simulink model "Tipo4_v4"  (R2018b)
settings: Solver=FixedStepDiscrete  StartTime=0.0  StopTime=50.3  MaxStep=50e-6  RelTol=1e-3
PreLoadFcn:
  | Ts=2e-6;
InitFcn:
  | %xInitial = init_power_wind_dfig_det;
  | Ts=2e-6;
undefined symbols (not defined in the file): D1, Delta, DiscIntNeverNeededParam, find_system
libraries: powerlib x144, simulink x110, powerlib_meascontrol x83, simulink_extras x6, powerlib_extras x4
(part 4 of 6)

== system Tipo4_v4/Subsystem7 ==
  In1 : Inport
  Bistable{,1..3} (4 alike) : powerlib_meascontrol/Logic/Bistable  Qpriority=Set  ic=0  Ts=Ts
      settings: SourceProductName=Simscape Power Systems  SourceProductBaseCode=PS
  Clock{,1..3} (4 alike) : Clock
  Compare To Constant{,2,4,6} (4 alike) : simulink/Logic and Bit Operations/Compare To Constant  relop=<=  const=100  OutDataTypeStr=uint8
  Compare To Constant1 : simulink/Logic and Bit Operations/Compare To Constant  relop=>=  const=Tini_FT  OutDataTypeStr=uint8
  Compare To Constant3 : simulink/Logic and Bit Operations/Compare To Constant  relop=>=  const=Tini_FF  OutDataTypeStr=uint8
  Compare To Constant5 : simulink/Logic and Bit Operations/Compare To Constant  relop=>=  const=Tini_FFT  OutDataTypeStr=uint8
  Compare To Constant7 : simulink/Logic and Bit Operations/Compare To Constant  relop=>=  const=Tini_FFF  OutDataTypeStr=uint8
  Compare To Constant8 : simulink/Logic and Bit Operations/Compare To Constant  relop=<=  const=0.1*pi/180  OutDataTypeStr=uint8
  Constant : Constant  Value=Tini_FT
  Constant1 : Constant  Value=Tini_FF
  Constant2 : Constant  Value=Tini_FFT
  Constant3 : Constant  Value=Tini_FFF
  Gain{,1..3} (4 alike) : Gain  OutDataTypeStr=double
  Ground : powerlib/Elements/Ground  LConnTagsString=a
  Ground1 : powerlib/Elements/Ground  LConnTagsString=a
  Ground2 : powerlib/Elements/Ground  LConnTagsString=a
  Mux1 : Mux  Inputs=3
  PLL (3ph) : powerlib_meascontrol/PLL/PLL (3ph)  Fmin=60  Par_Init=[0, 60]  ParK=[180, 3200, 1]  TcD=1e-4  MaxRateChangeFreq=12  FilterCutOffFreq=25  Ts=Ts  AGC=on
  Product{,2..7} (7 alike) : Product
  Product{1,8..11} (5 alike) : Product  RndMeth=Ceiling
  Scope{1..4} (4 alike) : Scope
  Three-Phase Fault1 : powerlib/Elements/Three-Phase Fault  InitialStates=0  FaultA=on  FaultB=off  FaultC=off  GroundFault=on  SwitchTimes=[900 1000]  External=on  SwitchStatus=NaN  FaultResistance=R_falta  GroundResistance=R_falta  SnubberResistance=1e6  SnubberCapacitance=inf  Measurements=None
  Three-Phase Fault2 : powerlib/Elements/Three-Phase Fault  InitialStates=0  FaultA=on  FaultB=on  FaultC=off  GroundFault=off  SwitchTimes=[900 1000]  External=on  SwitchStatus=NaN  FaultResistance=R_falta  GroundResistance=1e-12  SnubberResistance=1e6  SnubberCapacitance=inf  Measurements=None
  Three-Phase Fault3 : powerlib/Elements/Three-Phase Fault  InitialStates=0  FaultA=on  FaultB=on  FaultC=off  GroundFault=on  SwitchTimes=[900 1000]  External=on  SwitchStatus=NaN  FaultResistance=R_falta  GroundResistance=R_falta  SnubberResistance=1e6  SnubberCapacitance=inf  Measurements=None
  Three-Phase Fault4 : powerlib/Elements/Three-Phase Fault  InitialStates=0  FaultA=on  FaultB=on  FaultC=on  GroundFault=on  SwitchTimes=[900 1000]  External=on  SwitchStatus=NaN  FaultResistance=R_falta  GroundResistance=R_falta  SnubberResistance=1e6  SnubberCapacitance=inf  Measurements=None
  Voltage Measurement : powerlib/Measurements/Voltage Measurement  PhasorSimulation=off  OutputType=Complex  PSBequivalent=0
  Voltage Measurement1 : powerlib/Measurements/Voltage Measurement  PhasorSimulation=off  OutputType=Complex  PSBequivalent=0
  Voltage Measurement2 : powerlib/Measurements/Voltage Measurement  PhasorSimulation=off  OutputType=Complex  PSBequivalent=0
  A : PMIOPort  Tag=PMCPort  Side=Right
  B : PMIOPort  Tag=PMCPort  Port=2  Side=Right
  C : PMIOPort  Tag=PMCPort  Port=3  Side=Right
  wires:
  Clock/1 -> Compare To Constant1/1
  Product2/1 -> Product3/1
  Constant1/1 -> Compare To Constant2/1
  Product/1 -> Product1/1
  Compare To Constant2/1 -> Product2/2
  Constant2/1 -> Compare To Constant4/1
  Clock2/1 -> Compare To Constant5/1
  Compare To Constant4/1 -> Product4/2
  Clock1/1 -> Compare To Constant3/1
  Compare To Constant5/1 -> Product5/2
  In1/1 -> Product/1, Product2/1, Product4/1, Product6/1
  Clock3/1 -> Compare To Constant7/1
  Constant3/1 -> Compare To Constant6/1
  Compare To Constant6/1 -> Product6/2
  Product6/1 -> Product7/1
  Compare To Constant7/1 -> Product7/2
  Compare To Constant3/1 -> Product3/2
  Constant/1 -> Compare To Constant/1
  Compare To Constant/1 -> Product/2
  Compare To Constant1/1 -> Product1/2
  Product4/1 -> Product5/1
  Product1/1 -> Product8/2
  Product8/1 -> Bistable/1
  Product3/1 -> Product9/2
  Product5/1 -> Product10/2
  Product7/1 -> Product11/2
  Compare To Constant8/1 -> Product11/1, Product10/1, Product9/1, Product8/1
  PLL (3ph)/2 -> Compare To Constant8/1
  Voltage Measurement1/1 -> Mux1/2
  Voltage Measurement/1 -> Mux1/1
  Voltage Measurement2/1 -> Mux1/3
  Mux1/1 -> PLL (3ph)/1
  Gain/1 -> Scope1/1, Three-Phase Fault1/1
  Gain1/1 -> Scope2/1, Three-Phase Fault2/1
  Gain2/1 -> Three-Phase Fault3/1, Scope3/1
  Gain3/1 -> Scope4/1, Three-Phase Fault4/1
  Bistable/1 -> Gain/1
  Product9/1 -> Bistable1/1
  Bistable1/1 -> Gain1/1
  Bistable3/1 -> Gain2/1
  Product10/1 -> Bistable3/1
  Product11/1 -> Bistable2/1
  Bistable2/1 -> Gain3/1
  connections:
  Voltage Measurement1/LConn1 -- B/RConn1 -- Three-Phase Fault1/LConn2 -- Three-Phase Fault2/LConn2 -- Three-Phase Fault3/LConn2 -- Three-Phase Fault4/LConn2
  Voltage Measurement2/LConn1 -- C/RConn1 -- Three-Phase Fault4/LConn3 -- Three-Phase Fault3/LConn3 -- Three-Phase Fault2/LConn3 -- Three-Phase Fault1/LConn3
  A/RConn1 -- Voltage Measurement/LConn1 -- Three-Phase Fault1/LConn1 -- Three-Phase Fault2/LConn1 -- Three-Phase Fault3/LConn1 -- Three-Phase Fault4/LConn1
  Ground/LConn1 -- Voltage Measurement/LConn2
  Ground1/LConn1 -- Voltage Measurement1/LConn2
  Ground2/LConn1 -- Voltage Measurement2/LConn2

== system Tipo4_v4/Subsystem8 ==
  In1 : Inport
  Bistable{,1..3} (4 alike) : powerlib_meascontrol/Logic/Bistable  Qpriority=Set  ic=0  Ts=Ts
      settings: SourceProductName=Simscape Power Systems  SourceProductBaseCode=PS
  Clock{,1..3} (4 alike) : Clock
  Compare To Constant{,2,4,6} (4 alike) : simulink/Logic and Bit Operations/Compare To Constant  relop=<=  const=100  OutDataTypeStr=uint8
  Compare To Constant1 : simulink/Logic and Bit Operations/Compare To Constant  relop=>=  const=Tini_FT  OutDataTypeStr=uint8
  Compare To Constant3 : simulink/Logic and Bit Operations/Compare To Constant  relop=>=  const=Tini_FF  OutDataTypeStr=uint8
  Compare To Constant5 : simulink/Logic and Bit Operations/Compare To Constant  relop=>=  const=Tini_FFT  OutDataTypeStr=uint8
  Compare To Constant7 : simulink/Logic and Bit Operations/Compare To Constant  relop=>=  const=Tini_FFF  OutDataTypeStr=uint8
  Compare To Constant8 : simulink/Logic and Bit Operations/Compare To Constant  relop=<=  const=0.1*pi/180  OutDataTypeStr=uint8
  Constant : Constant  Value=Tini_FT
  Constant1 : Constant  Value=Tini_FF
  Constant2 : Constant  Value=Tini_FFT
  Constant3 : Constant  Value=Tini_FFF
  Gain{,1..3} (4 alike) : Gain  OutDataTypeStr=double
  Ground : powerlib/Elements/Ground  LConnTagsString=a
  Ground1 : powerlib/Elements/Ground  LConnTagsString=a
  Ground2 : powerlib/Elements/Ground  LConnTagsString=a
  Mux1 : Mux  Inputs=3
  PLL (3ph) : powerlib_meascontrol/PLL/PLL (3ph)  Fmin=60  Par_Init=[0, 60]  ParK=[180, 3200, 1]  TcD=1e-4  MaxRateChangeFreq=12  FilterCutOffFreq=25  Ts=Ts  AGC=on
  Product{,2..7} (7 alike) : Product
  Product{1,8..11} (5 alike) : Product  RndMeth=Ceiling
  Scope{1..4} (4 alike) : Scope
  Three-Phase Fault1 : powerlib/Elements/Three-Phase Fault  InitialStates=0  FaultA=on  FaultB=off  FaultC=off  GroundFault=on  SwitchTimes=[900 1000]  External=on  SwitchStatus=NaN  FaultResistance=R_falta  GroundResistance=R_falta  SnubberResistance=1e6  SnubberCapacitance=inf  Measurements=None
  Three-Phase Fault2 : powerlib/Elements/Three-Phase Fault  InitialStates=0  FaultA=on  FaultB=on  FaultC=off  GroundFault=off  SwitchTimes=[900 1000]  External=on  SwitchStatus=NaN  FaultResistance=R_falta  GroundResistance=1e-12  SnubberResistance=1e6  SnubberCapacitance=inf  Measurements=None
  Three-Phase Fault3 : powerlib/Elements/Three-Phase Fault  InitialStates=0  FaultA=on  FaultB=on  FaultC=off  GroundFault=on  SwitchTimes=[900 1000]  External=on  SwitchStatus=NaN  FaultResistance=R_falta  GroundResistance=R_falta  SnubberResistance=1e6  SnubberCapacitance=inf  Measurements=None
  Three-Phase Fault4 : powerlib/Elements/Three-Phase Fault  InitialStates=0  FaultA=on  FaultB=on  FaultC=on  GroundFault=on  SwitchTimes=[900 1000]  External=on  SwitchStatus=NaN  FaultResistance=R_falta  GroundResistance=R_falta  SnubberResistance=1e6  SnubberCapacitance=inf  Measurements=None
  Voltage Measurement : powerlib/Measurements/Voltage Measurement  PhasorSimulation=off  OutputType=Complex  PSBequivalent=0
  Voltage Measurement1 : powerlib/Measurements/Voltage Measurement  PhasorSimulation=off  OutputType=Complex  PSBequivalent=0
  Voltage Measurement2 : powerlib/Measurements/Voltage Measurement  PhasorSimulation=off  OutputType=Complex  PSBequivalent=0
  A : PMIOPort  Tag=PMCPort  Side=Right
  B : PMIOPort  Tag=PMCPort  Port=2  Side=Right
  C : PMIOPort  Tag=PMCPort  Port=3  Side=Right
  wires:
  Clock/1 -> Compare To Constant1/1
  Product2/1 -> Product3/1
  Constant1/1 -> Compare To Constant2/1
  Product/1 -> Product1/1
  Compare To Constant2/1 -> Product2/2
  Constant2/1 -> Compare To Constant4/1
  Clock2/1 -> Compare To Constant5/1
  Compare To Constant4/1 -> Product4/2
  Clock1/1 -> Compare To Constant3/1
  Compare To Constant5/1 -> Product5/2
  In1/1 -> Product/1, Product2/1, Product4/1, Product6/1
  Clock3/1 -> Compare To Constant7/1
  Constant3/1 -> Compare To Constant6/1
  Compare To Constant6/1 -> Product6/2
  Product6/1 -> Product7/1
  Compare To Constant7/1 -> Product7/2
  Compare To Constant3/1 -> Product3/2
  Constant/1 -> Compare To Constant/1
  Compare To Constant/1 -> Product/2
  Compare To Constant1/1 -> Product1/2
  Product4/1 -> Product5/1
  Product1/1 -> Product8/2
  Product8/1 -> Bistable/1
  Product3/1 -> Product9/2
  Product5/1 -> Product10/2
  Product7/1 -> Product11/2
  Compare To Constant8/1 -> Product11/1, Product10/1, Product9/1, Product8/1
  PLL (3ph)/2 -> Compare To Constant8/1
  Voltage Measurement1/1 -> Mux1/2
  Voltage Measurement/1 -> Mux1/1
  Voltage Measurement2/1 -> Mux1/3
  Mux1/1 -> PLL (3ph)/1
  Gain/1 -> Scope1/1, Three-Phase Fault1/1
  Gain1/1 -> Scope2/1, Three-Phase Fault2/1
  Gain2/1 -> Three-Phase Fault3/1, Scope3/1
  Gain3/1 -> Scope4/1, Three-Phase Fault4/1
  Bistable/1 -> Gain/1
  Product9/1 -> Bistable1/1
  Bistable1/1 -> Gain1/1
  Bistable3/1 -> Gain2/1
  Product10/1 -> Bistable3/1
  Product11/1 -> Bistable2/1
  Bistable2/1 -> Gain3/1
  connections:
  Voltage Measurement1/LConn1 -- B/RConn1 -- Three-Phase Fault1/LConn2 -- Three-Phase Fault2/LConn2 -- Three-Phase Fault3/LConn2 -- Three-Phase Fault4/LConn2
  Voltage Measurement2/LConn1 -- C/RConn1 -- Three-Phase Fault4/LConn3 -- Three-Phase Fault3/LConn3 -- Three-Phase Fault2/LConn3 -- Three-Phase Fault1/LConn3
  A/RConn1 -- Voltage Measurement/LConn1 -- Three-Phase Fault1/LConn1 -- Three-Phase Fault2/LConn1 -- Three-Phase Fault3/LConn1 -- Three-Phase Fault4/LConn1
  Ground/LConn1 -- Voltage Measurement/LConn2
  Ground1/LConn1 -- Voltage Measurement1/LConn2
  Ground2/LConn1 -- Voltage Measurement2/LConn2

== system Tipo4_v4/Subsystem9 ==
  In1 : Inport
  Bistable{,1..3} (4 alike) : powerlib_meascontrol/Logic/Bistable  Qpriority=Set  ic=0  Ts=Ts
      settings: SourceProductName=Simscape Power Systems  SourceProductBaseCode=PS
  Clock{,1..3} (4 alike) : Clock
  Compare To Constant{,2,4,6} (4 alike) : simulink/Logic and Bit Operations/Compare To Constant  relop=<=  const=100  OutDataTypeStr=uint8
  Compare To Constant1 : simulink/Logic and Bit Operations/Compare To Constant  relop=>=  const=Tini_FT  OutDataTypeStr=uint8
  Compare To Constant3 : simulink/Logic and Bit Operations/Compare To Constant  relop=>=  const=Tini_FF  OutDataTypeStr=uint8
  Compare To Constant5 : simulink/Logic and Bit Operations/Compare To Constant  relop=>=  const=Tini_FFT  OutDataTypeStr=uint8
  Compare To Constant7 : simulink/Logic and Bit Operations/Compare To Constant  relop=>=  const=Tini_FFF  OutDataTypeStr=uint8
  Compare To Constant8 : simulink/Logic and Bit Operations/Compare To Constant  relop=<=  const=0.1*pi/180  OutDataTypeStr=uint8
  Constant : Constant  Value=Tini_FT
  Constant1 : Constant  Value=Tini_FF
  Constant2 : Constant  Value=Tini_FFT
  Constant3 : Constant  Value=Tini_FFF
  Gain{,1..3} (4 alike) : Gain  OutDataTypeStr=double
  Ground : powerlib/Elements/Ground  LConnTagsString=a
  Ground1 : powerlib/Elements/Ground  LConnTagsString=a
  Ground2 : powerlib/Elements/Ground  LConnTagsString=a
  Mux1 : Mux  Inputs=3
  PLL (3ph) : powerlib_meascontrol/PLL/PLL (3ph)  Fmin=60  Par_Init=[0, 60]  ParK=[180, 3200, 1]  TcD=1e-4  MaxRateChangeFreq=12  FilterCutOffFreq=25  Ts=Ts  AGC=on
  Product{,2..7} (7 alike) : Product
  Product{1,8..11} (5 alike) : Product  RndMeth=Ceiling
  Scope{1..4} (4 alike) : Scope
  Three-Phase Fault1 : powerlib/Elements/Three-Phase Fault  InitialStates=0  FaultA=on  FaultB=off  FaultC=off  GroundFault=on  SwitchTimes=[900 1000]  External=on  SwitchStatus=NaN  FaultResistance=R_falta  GroundResistance=R_falta  SnubberResistance=1e6  SnubberCapacitance=inf  Measurements=None
  Three-Phase Fault2 : powerlib/Elements/Three-Phase Fault  InitialStates=0  FaultA=on  FaultB=on  FaultC=off  GroundFault=off  SwitchTimes=[900 1000]  External=on  SwitchStatus=NaN  FaultResistance=R_falta  GroundResistance=1e-12  SnubberResistance=1e6  SnubberCapacitance=inf  Measurements=None
  Three-Phase Fault3 : powerlib/Elements/Three-Phase Fault  InitialStates=0  FaultA=on  FaultB=on  FaultC=off  GroundFault=on  SwitchTimes=[900 1000]  External=on  SwitchStatus=NaN  FaultResistance=R_falta  GroundResistance=R_falta  SnubberResistance=1e6  SnubberCapacitance=inf  Measurements=None
  Three-Phase Fault4 : powerlib/Elements/Three-Phase Fault  InitialStates=0  FaultA=on  FaultB=on  FaultC=on  GroundFault=on  SwitchTimes=[900 1000]  External=on  SwitchStatus=NaN  FaultResistance=R_falta  GroundResistance=R_falta  SnubberResistance=1e6  SnubberCapacitance=inf  Measurements=None
  Voltage Measurement : powerlib/Measurements/Voltage Measurement  PhasorSimulation=off  OutputType=Complex  PSBequivalent=0
  Voltage Measurement1 : powerlib/Measurements/Voltage Measurement  PhasorSimulation=off  OutputType=Complex  PSBequivalent=0
  Voltage Measurement2 : powerlib/Measurements/Voltage Measurement  PhasorSimulation=off  OutputType=Complex  PSBequivalent=0
  A : PMIOPort  Tag=PMCPort  Side=Right
  B : PMIOPort  Tag=PMCPort  Port=2  Side=Right
  C : PMIOPort  Tag=PMCPort  Port=3  Side=Right
  wires:
  Clock/1 -> Compare To Constant1/1
  Product2/1 -> Product3/1
  Constant1/1 -> Compare To Constant2/1
  Product/1 -> Product1/1
  Compare To Constant2/1 -> Product2/2
  Constant2/1 -> Compare To Constant4/1
  Clock2/1 -> Compare To Constant5/1
  Compare To Constant4/1 -> Product4/2
  Clock1/1 -> Compare To Constant3/1
  Compare To Constant5/1 -> Product5/2
  In1/1 -> Product/1, Product2/1, Product4/1, Product6/1
  Clock3/1 -> Compare To Constant7/1
  Constant3/1 -> Compare To Constant6/1
  Compare To Constant6/1 -> Product6/2
  Product6/1 -> Product7/1
  Compare To Constant7/1 -> Product7/2
  Compare To Constant3/1 -> Product3/2
  Constant/1 -> Compare To Constant/1
  Compare To Constant/1 -> Product/2
  Compare To Constant1/1 -> Product1/2
  Product4/1 -> Product5/1
  Product1/1 -> Product8/2
  Product8/1 -> Bistable/1
  Product3/1 -> Product9/2
  Product5/1 -> Product10/2
  Product7/1 -> Product11/2
  Compare To Constant8/1 -> Product11/1, Product10/1, Product9/1, Product8/1
  PLL (3ph)/2 -> Compare To Constant8/1
  Voltage Measurement1/1 -> Mux1/2
  Voltage Measurement/1 -> Mux1/1
  Voltage Measurement2/1 -> Mux1/3
  Mux1/1 -> PLL (3ph)/1
  Gain/1 -> Scope1/1, Three-Phase Fault1/1
  Gain1/1 -> Scope2/1, Three-Phase Fault2/1
  Gain2/1 -> Three-Phase Fault3/1, Scope3/1
  Gain3/1 -> Scope4/1, Three-Phase Fault4/1
  Bistable/1 -> Gain/1
  Product9/1 -> Bistable1/1
  Bistable1/1 -> Gain1/1
  Bistable3/1 -> Gain2/1
  Product10/1 -> Bistable3/1
  Product11/1 -> Bistable2/1
  Bistable2/1 -> Gain3/1
  connections:
  Voltage Measurement1/LConn1 -- B/RConn1 -- Three-Phase Fault1/LConn2 -- Three-Phase Fault2/LConn2 -- Three-Phase Fault3/LConn2 -- Three-Phase Fault4/LConn2
  Voltage Measurement2/LConn1 -- C/RConn1 -- Three-Phase Fault4/LConn3 -- Three-Phase Fault3/LConn3 -- Three-Phase Fault2/LConn3 -- Three-Phase Fault1/LConn3
  A/RConn1 -- Voltage Measurement/LConn1 -- Three-Phase Fault1/LConn1 -- Three-Phase Fault2/LConn1 -- Three-Phase Fault3/LConn1 -- Three-Phase Fault4/LConn1
  Ground/LConn1 -- Voltage Measurement/LConn2
  Ground1/LConn1 -- Voltage Measurement1/LConn2
  Ground2/LConn1 -- Voltage Measurement2/LConn2

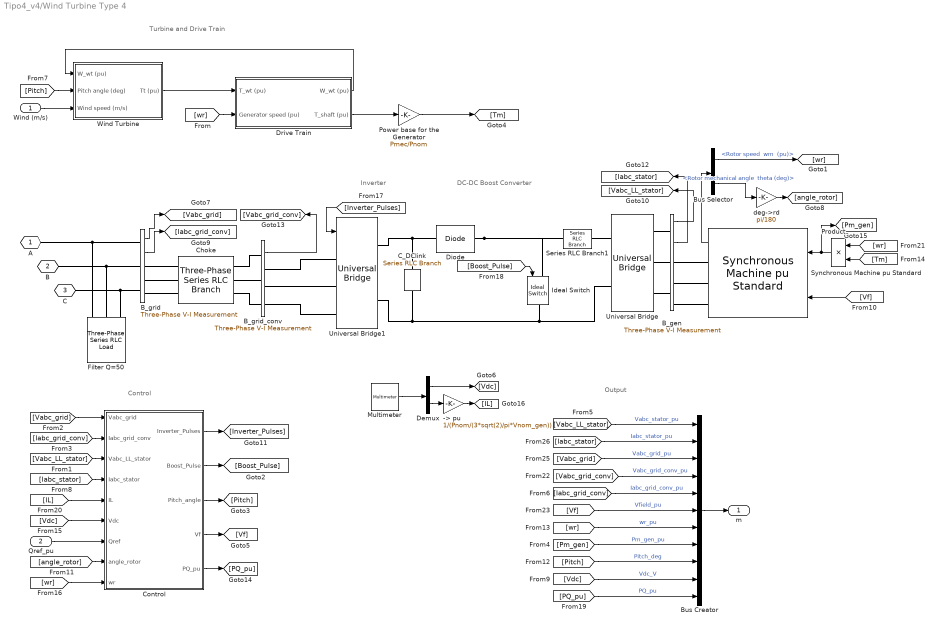
== system Tipo4_v4/Wind Turbine Type 4 ==
  note: Turbine and Drive Train
  note: Control
  note: Inverter
  note: DC-DC Boost Converter
  note: Output
  "Wind (m/s) " : Inport
  Qref_pu : Inport  Port=2
  -> pu : Gain  Gain=1/(Pnom/(3*sqrt(2)/pi*Vnom_gen))  SaturateOnIntegerOverflow=on  OutDataTypeStr=Inherit: Same as input  ParamDataTypeStr=Inherit: Same as input
  B_gen : powerlib/Measurements/Three-Phase V-I Measurement  VoltageMeasurement=phase-to-phase  SetLabelV=off  LabelV=Vabc  Vpu=on  VpuLL=off  CurrentMeasurement=yes  SetLabelI=off  LabelI=Iabc  Ipu=on  Pbase=Pnom  Vbase=Vnom_gen  OutputType=Complex  PhasorSimulation=off  PSBequivalent=0
      settings: SourceProductName=Simscape Electrical
  B_grid : powerlib/Measurements/Three-Phase V-I Measurement  VoltageMeasurement=phase-to-ground  SetLabelV=off  LabelV=Vabc  Vpu=on  VpuLL=off  CurrentMeasurement=yes  SetLabelI=off  LabelI=Iabc  Ipu=on  Pbase=Pnom  Vbase=Vnom  OutputType=Complex  PhasorSimulation=off  PSBequivalent=0
      settings: SourceProductName=Simscape Electrical
  B_grid_conv : powerlib/Measurements/Three-Phase V-I Measurement  VoltageMeasurement=phase-to-ground  SetLabelV=off  LabelV=Vabc  Vpu=on  VpuLL=off  CurrentMeasurement=no  SetLabelI=off  LabelI=Iabc  Ipu=on  Pbase=Pnom  Vbase=Vnom  OutputType=Complex  PhasorSimulation=off  PSBequivalent=0
      settings: SourceProductName=Simscape Electrical
  Bus Creator : BusCreator  Inputs=11
  Bus Selector : BusSelector  OutputSignals="Mechanical.Rotor speed  wm  (pu),Mechanical.Rotor mechanical angle  theta (deg)"
  C_DClink : powerlib/Elements/Series RLC Branch  LConnTagsString=__new0  RConnTagsString=__new0  BranchType=C  Resistance=1  Inductance=1e-3  SetiL0=off  InitialCurrent=0  Capacitance=C_DClink  Setx0=on  InitialVoltage=Vdc_nom  Measurements=Branch voltage
      settings: SourceProductName=Simscape Electrical
  "Choke " : powerlib/Elements/Three-Phase Series RLC Branch  LConnTagsString=A|B|C  RConnTagsString=A|B|C  BranchType=RL  Resistance=R_RL*Vnom^2/Pnom  Inductance=L_RL*Vnom^2/Pnom/(2*pi*Fnom)  Capacitance=[]  Measurements=None
      settings: SourceProductName=Simscape Electrical
  Control : Subsystem
  Demux : Demux  Outputs=2
  Diode : powerlib/Power Electronics/Diode  Ron=1e-6/Nb_wt  Lon=0  Vf=0  IC=0  UseSnubber=off  Rs=inf  Cs=inf  Measurements=off
      settings: SourceProductName=Simscape Electrical
  Drive Train : Subsystem  mask(Wind Turbine shaft){H_WT=H_WT, Ksh=Ksh, D_mutual=D_mutual, wbase=2*pi*Fnom/p, w_wt0=w_wt0, torque0=torque0, Ts=Ts}
      mask prompts: H_WT "Wind turbine inertia constant H (s):"; Ksh "Shaft spring constant (pu of nominal mechanical torque/rad):"; D_mutual "Shaft mutual damping (pu of nominal mechanical torque/pu dw):"; wbase "Shaft base speed (rad/s):"; w_wt0 "Turbine initial speed (pu of base speed):"; torque0 "Initial output torque (pu of nominal mechanical torque):"; Ts "Sample time (s):"
      mask help:
      | This block implements a wind turbine drive train model. All shaft parameters are referred to high-speed shaft (generator shaft).
      |
      | The first input is the wind turbine torque in per unit (pu) based on the nominal power of the turbine and the base speed of the generator. The second input is the generator speed in pu based on the base speed of the generator.
      |
      | The outputs are:
      | 1- the transmitted torque of the shaft in pu based on the nominal power of the turbine and the base speed of the generator.
      | 2- the wind turbine speed in pu of the base speed of the generator.
  Filter Q=50 : powerlib/Elements/Three-Phase Series RLC Load  LConnTagsString=A|B|C  Configuration=Y (grounded)  NominalVoltage=Vnom  Vabc=[1e3 1e3 1e3]  Vabcp=[1e3 1e3 1e3]  NominalFrequency=Fnom  UnbalancedPower=off  ActivePower=C_var_filter/Q_filter  InductivePower=0  CapacitivePower=C_var_filter  Pabc=[10e3 9e3 11e3]  QLabc=[100 90 110]  QCabc=[100 90 110]  Pabcp=[10e3 9e3 11e3]  QLabcp=[100 90 110]  QCabcp=[100 90 110]  Measurements=None  LoadType=constant Z
      settings: SourceProductName=Simscape Electrical
  Ideal Switch : powerlib/Power Electronics/Ideal Switch  Ron=1e-6/Nb_wt  Lon=0  IC=0  Rs=1e5/Nb_wt  Cs=inf  Measurements=off
      settings: SourceProductName=Simscape Electrical
  Multimeter : powerlib/Measurements/Multimeter  PhasorSimulation=off  OutputType=Complex  sel=[1 2]  L=2  Gain=[1 1]  yselected={'Ub: Wind Turbine Type 4/C_DClink','Ib: Wind Turbine Type 4/Series RLC Branch1'};  PSBOutputType=1  PSBequivalent=0  AxesSetting=[0,0.1,-100,100]  Display=0  SavedBlockNames=-11
      settings: SourceProductName=Simscape Electrical
  Power base for the Generator : Gain  Gain=Pmec/Pnom  SaturateOnIntegerOverflow=on  OutDataTypeStr=Inherit: Same as input  ParamDataTypeStr=Inherit: Same as input
  Product : Product  RndMeth=Zero
  Series RLC Branch1 : powerlib/Elements/Series RLC Branch  LConnTagsString=__new0  RConnTagsString=__new0  BranchType=RL  Resistance=R_Boost  Inductance=L_Boost  SetiL0=off  InitialCurrent=0  Capacitance=1.0  Setx0=off  InitialVoltage=0  Measurements=Branch current
      settings: SourceProductName=Simscape Electrical
  Synchronous Machine pu Standard : powerlib/Machines/Synchronous Machine pu Standard  PresetModel=No  MechanicalLoad=Mechanical power Pm  ShowDetailedParameters=on  RotorType=Salient-pole  Units=per unit standard parameters  MeasurementBus=off  NominalParameters="[ Pnom  Vnom_gen Fnom ]"  Reactances1=[ 1.81, 0.3, 0.23, 1.76, 0.65, 0.25, 0.15 ]  Reactances2="[ Xd, Xd1, Xd2, Xq,  Xq2,  Xl ]"  dAxisTimeConstants=Open-circuit  qAxisTimeConstants=Short-circuit  TimeConstants1="[ 4.4849  0.0681  0.1  ]"  TimeConstants2=[ 8.0, 0.03, 1.0, 0.07 ]  TimeConstants3="[  Tdo1  Tdo2  Tq2  ]"  TimeConstants4=[ 8.0, 0.03, 0.3371, 0.0295 ]  TimeConstants5=[ 1.01, 0.053, 0.1 ]  TimeConstants6=[ 1.3201, 0.023, 1.0, 0.07 ]  TimeConstants7="[  1.01  0.053  0.051266  ]"  TimeConstants8=[ 1.3201, 0.0231, 0.3371, 0.0295 ]  StatorResistance=Resistance  Mechanical=[ H F p]  PolePairs=1  InitialConditions=init  SetSaturation=off  Saturation=[0.6404,0.7127,0.8441,0.9214,0.9956,1.082,1.19,1.316,1.457;0.7,0.7698,0.8872,0.9466,0.9969,1.046,1.1,1.151,1.201]  LoadFlowParameters=[1,0,0,0,0]  TsPowergui=0  TsBlock=-1  IterativeModel=Trapezoidal non iterative  IterativeDiscreteModel=Trapezoidal non iterative  BusType=PV  Pref=0  Qref=0  Qmin=-inf  Qmax=inf  PLF=0  QLF=0
      settings: SourceProductName=Simscape Electrical
  Universal Bridge : powerlib/Power Electronics/Universal Bridge  Arms=3  SnubberResistance=2*Ts_snub/(Pnom/(1000*2*pi*Fnom*Vnom_gen^2))  SnubberCapacitance=Pnom/(1000*2*pi*Fnom*Vnom_gen^2)  Device=Diodes  Ron=1e-6/Nb_wt  Lon=0  ForwardVoltages="[  0  0  ]"  ForwardVoltage=0  GTOparameters=[ 10e-6 , 20e-6 ]  IGBTparameters=[ 1e-6 , 2e-6 ]  Measurements=None  Measurements_2=None  converterType=Rectifier
      settings: SourceProductName=Simscape Electrical
  Universal Bridge1 : powerlib/Power Electronics/Universal Bridge  Arms=3  SnubberResistance=1e6/Nb_wt  SnubberCapacitance=inf  Device=IGBT / Diodes  Ron=1e-6/Nb_wt  Lon=0  ForwardVoltages="[  0  0  ]"  ForwardVoltage=0  GTOparameters=[ 10e-6 , 20e-6 ]  IGBTparameters=[ 1e-6 , 2e-6 ]*0  Measurements=None  Measurements_2=None  converterType=Rectifier
      settings: SourceProductName=Simscape Electrical
  Wind Turbine : Subsystem  mask(Wind Turbine){Prated=Pmec, c1_c8=c1_c8, K1_K2=K1_K2, wind0=wind0, Ts=Ts}
      mask prompts: Prated "Nominal mechanical output power (W):"; c1_c8 "Coefficients [c1 ... c8]"; K1_K2 "Parameters [K1 K2]"; wind0 "Initial wind speed (m/s):"; Ts "Sample time (s):"
      mask help:
      | This block implements a generic wind turbine models.
      |
      | The first input is the turbine speed in per unit of the generator base speed. For a synchronous or asynchronous generator, the base speed is the synchronous speed. For a permanent-magnet generator, the base speed is defined as the speed producing nominal voltage at  no load. The second input is the blade pitch angle in degrees. The third input is the wind speed in m/s.
      |
      | The output is the torque applied to the drive train in per unit based on the nominal power of the turbine and the base speed of the generator.
      mask init:
      | c1 = c1_c8(1);
      | c2 = c1_c8(2);
      | c3 = c1_c8(3);
      | c4 = c1_c8(4);
      | c5 = c1_c8(5);
      | c6 = c1_c8(6);
      | c7 = c1_c8(7);;
      | c8 = c1_c8(8);
      | 
      | K1=K1_K2(1);
      | K2=K1_K2(2);
      settings: OpenFcn=power_openblockproxy();
      mask Display: disp('');
  deg->rd : Gain  Gain=pi/180  SaturateOnIntegerOverflow=on  OutDataTypeStr=Inherit: Same as input  ParamDataTypeStr=Inherit: Same as input
  A : PMIOPort  Tag=PMCPort  Side=Left
  B : PMIOPort  Tag=PMCPort  Port=2  Side=Left
  C : PMIOPort  Tag=PMCPort  Port=3  Side=Left
  m : Outport
  wires:
  [Vf] -> Synchronous Machine pu Standard/2
  Wind Turbine/1(Tt (pu)) -> Drive Train/1(T_wt (pu))
  [wr] -> Drive Train/2(Generator speed (pu))
  Drive Train/2(T_shaft (pu)) -> Power base for the Generator/1
  Power base for the Generator/1 -> [Tm]
  "Wind (m/s) "/1 -> Wind Turbine/3(Wind speed (m/s))
  Drive Train/1(W_wt (pu)) -> Wind Turbine/1(W_wt (pu))
  [Pitch] -> Wind Turbine/2(Pitch angle (deg))
  Bus Selector/2 -> deg->rd/1  "<Rotor mechanical angle  theta (deg)>"
  deg->rd/1 -> [angle_rotor]
  Bus Selector/1 -> [wr]  "<Rotor speed  wm  (pu)>"
  [wr] -> Product/1
  Synchronous Machine pu Standard/1 -> Bus Selector/1
  B_grid_conv/1 -> [Vabc_grid_conv]
  [Tm] -> Product/2
  Product/1 -> Synchronous Machine pu Standard/1, [Pm_gen]
  B_grid/1 -> [Vabc_grid]
  B_grid/2 -> [Iabc_grid_conv]
  B_gen/1 -> [Vabc_LL_stator]
  B_gen/2 -> [Iabc_stator]
  [Vabc_grid] -> Control/1(Vabc_grid)
  [Iabc_grid_conv] -> Control/2(Iabc_grid_conv)
  [Vabc_LL_stator] -> Control/3(Vabc_LL_stator)
  [Iabc_stator] -> Control/4(Iabc_stator)
  [Vdc] -> Control/6(Vdc)
  Qref_pu/1 -> Control/7(Qref)
  [angle_rotor] -> Control/8(angle_rotor)
  [wr] -> Control/9(wr)
  Control/1(Inverter_Pulses) -> [Inverter_Pulses]
  Control/2(Boost_Pulse) -> [Boost_Pulse]
  Control/3(Pitch_angle) -> [Pitch]
  Control/4(Vf) -> [Vf]
  [Inverter_Pulses] -> Universal Bridge1/1
  [Boost_Pulse] -> Ideal Switch/1
  Control/5(PQ_pu) -> [PQ_pu]
  [Vabc_LL_stator] -> Bus Creator/1  "Vabc_stator_pu"
  [Iabc_stator] -> Bus Creator/2  "Iabc_stator_pu"
  [Vabc_grid] -> Bus Creator/3  "Vabc_grid_pu"
  Bus Creator/1 -> m/1
  [Vabc_grid_conv] -> Bus Creator/4  "Vabc_grid_conv_pu"
  [Iabc_grid_conv] -> Bus Creator/5  "Iabc_grid_conv_pu"
  [Vf] -> Bus Creator/6  "Vfield_pu"
  [wr] -> Bus Creator/7  "wr_pu"
  [Pm_gen] -> Bus Creator/8  "Pm_gen_pu"
  [Pitch] -> Bus Creator/9  "Pitch_deg"
  [Vdc] -> Bus Creator/10  "Vdc_V"
  [PQ_pu] -> Bus Creator/11  "PQ_pu"
  [IL] -> Control/5(IL)
  Multimeter/1 -> Demux/1
  Demux/1 -> [Vdc]
  Demux/2 -> -> pu/1
  -> pu/1 -> [IL]
  connections:
  B_grid/RConn1 -- "Choke "/LConn1
  B_grid/RConn2 -- "Choke "/LConn2
  B_grid/RConn3 -- "Choke "/LConn3
  A/RConn1 -- B_grid/LConn1 -- Filter Q=50/LConn1
  Filter Q=50/LConn2 -- B_grid/LConn2 -- B/RConn1
  Filter Q=50/LConn3 -- B_grid/LConn3 -- C/RConn1
  "Choke "/RConn1 -- B_grid_conv/LConn1
  "Choke "/RConn2 -- B_grid_conv/LConn2
  "Choke "/RConn3 -- B_grid_conv/LConn3
  Series RLC Branch1/LConn1 -- Universal Bridge/RConn1
  Universal Bridge/LConn1 -- B_gen/LConn1
  Universal Bridge/LConn2 -- B_gen/LConn2
  Universal Bridge/LConn3 -- B_gen/LConn3
  Diode/LConn1 -- Series RLC Branch1/RConn1 -- Ideal Switch/LConn1
  Universal Bridge1/RConn1 -- Diode/RConn1 -- C_DClink/LConn1
  Universal Bridge/RConn2 -- Universal Bridge1/RConn2 -- C_DClink/RConn1 -- Ideal Switch/RConn1
  Synchronous Machine pu Standard/RConn3 -- B_gen/RConn3
  Synchronous Machine pu Standard/RConn2 -- B_gen/RConn2
  Synchronous Machine pu Standard/RConn1 -- B_gen/RConn1
  B_grid_conv/RConn2 -- Universal Bridge1/LConn2
  B_grid_conv/RConn1 -- Universal Bridge1/LConn1
  B_grid_conv/RConn3 -- Universal Bridge1/LConn3

== system Tipo4_v4/Wind Turbine Type 4/Control ==
  note: Inputs
  note: Grid-Side Converter
      | Control System
  note: Speed Regulator & Pitch Control
  note: Excitation
      | Control system
  Vabc_grid : Inport
  Iabc_grid_conv : Inport  Port=2
  Vabc_LL_stator : Inport  Port=3
  Iabc_stator : Inport  Port=4
  IL : Inport  Port=5
  Vdc : Inport  Port=6
  Qref : Inport  Port=7
  angle_rotor : Inport  Port=8
  wr : Inport  Port=9
  Bus Creator : BusCreator  Inputs=2
  Excitation Control system : Subsystem
  Grid-side converter Control system : Subsystem
  Measurement and Transformation : Subsystem
  PWM Generator (2-Level) : powerlib_meascontrol/Pulse & Signal Generators/PWM Generator (2-Level)  ModulatorType=Three-phase bridge (6 pulses)  ModulatorMode=Unsynchronized  Fc=Freq_PWM  Pc=90  nF=27  MinMax="[ -1  1 ]"  SamplingTechnique=Natural  ModulatingSignals=off  m=0.8  Freq=60  Phase=0  Ts=Ts  ShowCarrierOutport=off
  Pulse Generator : Subsystem  mask{Freq_sawtooth=Freq_sawtooth, Ts=Ts}
      mask prompts: Freq_sawtooth "Frequency of the carrier (sawtooth signal) (Hz):"; Ts "Sample time (Ts) (s):"
  Speed & Pitch Control : Subsystem
  Unit Delay{1..4,6..7} (6 alike) : UnitDelay  SampleTime=Ts
  Inverter_Pulses : Outport
  Boost_Pulse : Outport  Port=2
  Pitch_angle : Outport  Port=3
  Vf : Outport  Port=4
  PQ_pu : Outport  Port=5
  wires:
  Excitation Control system/1(Vf) -> Unit Delay4/1
  Speed & Pitch Control/2(Pitch (deg)) -> Unit Delay1/1
  [Idq_gc] -> Grid-side converter Control system/1(Idq_gc)
  [w_pu] -> Grid-side converter Control system/2(w_pu)
  [Vdq_grid] -> Grid-side converter Control system/3(Vdq_grid)
  [Vdc_meas] -> Grid-side converter Control system/4(Vdc)
  [Qref] -> Grid-side converter Control system/5(Qref)
  [Qmeas] -> Grid-side converter Control system/6(Qmeas)
  [Vmeas] -> Grid-side converter Control system/7(Vmeas)
  Speed & Pitch Control/1(Duty_Cycle) -> Unit Delay2/1
  [Flux] -> Excitation Control system/1(Flux)
  [wr] -> Excitation Control system/2(wr)
  [Theta_PLL] -> Grid-side converter Control system/8(Theta_PLL)
  Unit Delay2/1 -> Pulse Generator/1(Duty_Cycle)
  Unit Delay1/1 -> Pitch_angle/1
  Unit Delay4/1 -> Vf/1
  PWM Generator (2-Level)/1 -> Inverter_Pulses/1
  Grid-side converter Control system/1(Uctrl_inverter) -> Unit Delay6/1
  Pulse Generator/1(Pulse) -> Boost_Pulse/1
  Unit Delay6/1 -> PWM Generator (2-Level)/1
  Bus Creator/1 -> PQ_pu/1
  [Pmeas] -> Unit Delay3/1
  [Qmeas] -> Unit Delay7/1
  Unit Delay3/1 -> Bus Creator/1  "P_pu"
  Unit Delay7/1 -> Bus Creator/2  "Q_pu"
  [wr] -> Speed & Pitch Control/1(wr)
  [Pmeas] -> Speed & Pitch Control/2(Pmeas)
  [IL] -> Speed & Pitch Control/3(IL)
  Vabc_grid/1 -> Measurement and Transformation/1(Vabc_grid)
  Iabc_grid_conv/1 -> Measurement and Transformation/2(Iabc_gc)
  Vabc_LL_stator/1 -> Measurement and Transformation/3(Vabc_LL_s)
  Iabc_stator/1 -> Measurement and Transformation/4(Iabc_s)
  IL/1 -> Measurement and Transformation/5(IL)
  Vdc/1 -> Measurement and Transformation/6(Vdc)
  Qref/1 -> Measurement and Transformation/7(Qref)
  angle_rotor/1 -> Measurement and Transformation/8(angle_rotor)
  wr/1 -> Measurement and Transformation/9(wr)
  Measurement and Transformation/1(Vdq_grid) -> [Vdq_grid]
  Measurement and Transformation/2(Idq_gc) -> [Idq_gc]
  Measurement and Transformation/3("IL ") -> [IL]
  Measurement and Transformation/4(Flux) -> [Flux]
  Measurement and Transformation/5(Vdc_meas) -> [Vdc_meas]
  Measurement and Transformation/6(Pmeas) -> [Pmeas]
  Measurement and Transformation/7(Qmeas) -> [Qmeas]
  Measurement and Transformation/8(Vmeas) -> [Vmeas]
  Measurement and Transformation/9(Theta_PLL) -> [Theta_PLL]
  Measurement and Transformation/10(w_pu) -> [w_pu]
  Measurement and Transformation/11("wr ") -> [wr]
  Measurement and Transformation/12("Qref ") -> [Qref]

== system Tipo4_v4/Wind Turbine Type 4/Drive Train ==
  note: Wind turbine drive train based on a 2-masse model
  note: Turbine
  note: Shaft
  T_wt (pu) : Inport
  Generator speed (pu) : Inport  Port=2
  1_2H_WT : Gain  Gain=1/(2*H_WT)  SaturateOnIntegerOverflow=on  OutDataTypeStr=Inherit: Same as input  ParamDataTypeStr=Inherit: Same as input
  Discrete-Time Integrator : DiscreteIntegrator  InitialCondition=w_wt0  SampleTime=Ts  ICPrevOutput=DiscIntNeverNeededParam  ICPrevScaledInput=DiscIntNeverNeededParam
  Discrete-Time Integrator1 : DiscreteIntegrator  InitialCondition=torque0/Ksh  SampleTime=Ts  ICPrevOutput=DiscIntNeverNeededParam  ICPrevScaledInput=DiscIntNeverNeededParam
  Mutual damping : Gain  Gain=D_mutual  SaturateOnIntegerOverflow=on  OutDataTypeStr=Inherit: Same as input  ParamDataTypeStr=Inherit: Same as input
  Stiffness : Gain  Gain=Ksh  SaturateOnIntegerOverflow=on  OutDataTypeStr=Inherit: Same as input  ParamDataTypeStr=Inherit: Same as input
  Sum : Sum  Inputs=+-  SaturateOnIntegerOverflow=on  InputSameDT=on  OutDataTypeStr=Inherit: Same as first input
  Sum1 : Sum  Inputs=+-  SaturateOnIntegerOverflow=on  InputSameDT=on  OutDataTypeStr=Inherit: Same as first input
  Sum2 : Sum  SaturateOnIntegerOverflow=on  InputSameDT=on  OutDataTypeStr=Inherit: Same as first input
  wbase : Gain  Gain=wbase  SaturateOnIntegerOverflow=on  OutDataTypeStr=Inherit: Same as input  ParamDataTypeStr=Inherit: Same as input
  W_wt (pu) : Outport
  T_shaft (pu) : Outport  Port=2
  wires:
  T_wt (pu)/1 -> Sum/1
  Sum2/1 -> T_shaft (pu)/1, Sum/2
  Mutual damping/1 -> Sum2/2
  Sum1/1 -> Mutual damping/1, wbase/1
  Generator speed (pu)/1 -> Sum1/2
  Discrete-Time Integrator/1 -> W_wt (pu)/1, Sum1/1
  1_2H_WT/1 -> Discrete-Time Integrator/1
  Sum/1 -> 1_2H_WT/1
  Stiffness/1 -> Sum2/1
  Discrete-Time Integrator1/1 -> Stiffness/1
  wbase/1 -> Discrete-Time Integrator1/1

== system Tipo4_v4/Wind Turbine Type 4/Wind Turbine ==
  W_wt (pu) : Inport
  Pitch angle (deg) : Inport  Port=2
  Wind speed (m/s) : Inport  Port=3
  ->pu : Gain  Gain=1/Prated
  Avoid div. by zero : Saturate  UpperLimit=inf  LowerLimit=eps
  "Avoid div. by zero " : Saturate  UpperLimit=inf  LowerLimit=eps
  Fcn1 : Fcn  Expr=K1*u[2]/u[1]
  Fcn2 : Fcn  Expr=c1*(c6*u[1] + (-c4 - c3*(2.5 + u[2]) + c2*(1/(u[1] + c7*(2.5 + u[2])) -c8/(1 + (2.5 + u[2])^3)))/exp(c5*(1/(u[1] + c7*(2.5 + u[2])) - c8/(1 + (2.5 + u[2])^3))))
  "K2*Cp*wind^3 " : Fcn  Expr=K2*u[1]^3*u[2]
  Mux : Mux  Inputs=2
  Mux1 : Mux  Inputs=2
  Mux2 : Mux  Inputs=2
  Product2 : Product  Inputs=*/  SaturateOnIntegerOverflow=on  InputSameDT=on  OutDataTypeStr=Inherit: Same as first input
  Tt (pu) : Outport
  wires:
  ->pu/1 -> Product2/1  "power_pu"
  Product2/1 -> Tt (pu)/1
  Wind speed (m/s)/1 -> Avoid div. by zero/1
  Fcn1/1 -> Mux1/1  "lambda"
  Mux1/1 -> Fcn2/1
  Mux/1 -> Fcn1/1
  Fcn2/1 -> Mux2/2  "Cp"
  Mux2/1 -> "K2*Cp*wind^3 "/1
  Pitch angle (deg)/1 -> Mux1/2
  W_wt (pu)/1 -> "Avoid div. by zero "/1
  Avoid div. by zero/1 -> Mux2/1, Mux/1
  "Avoid div. by zero "/1 -> Mux/2, Product2/2
  "K2*Cp*wind^3 "/1 -> ->pu/1

== system Tipo4_v4/Wind Turbine Type 4/Control/Excitation Control system ==
  Flux : Inport
  wr : Inport  Port=2
  Discrete PI Controller : Subsystem  DialogController=POWERSYS.PowerSysDialog  mask(Discrete PI Controller){Kp=Kp_field, Ki=Ki_field, Par_Limits=[1 0]*Vf_limit, Init=init(9), Ts=Ts}
      mask prompts: Kp "Proportional gain (Kp):"; Ki "Integral gain (Ki):"; Par_Limits "Output limits: [ Upper   Lower ]"; Init "Output initial value:"; Ts "Sample time:"
      mask help: This block implements a discrete PI controller.
      mask init:
      | UpperLimit=Par_Limits(1);
      | LowerLimit=Par_Limits(2);
      | power_initmask();
      mask Help: This block is part of a subset of blocks in the Extras library that does not have documentation associated with it, other than the block mask description.
      mask Display: disp('PI');
  Divide : Product  Inputs=*/
  Flux_ref : Constant
  "Flux_ref " : Constant
  Sum4 : Sum  Inputs=|+-  SaturateOnIntegerOverflow=on  InputSameDT=on  OutDataTypeStr=Inherit: Same as first input
  Switch : Switch  Threshold=1
  avoid division by 0 : Saturate  UpperLimit=inf  LowerLimit=1e-6
  Vf : Outport
  wires:
  Switch/1 -> Sum4/1
  Divide/1 -> Switch/1
  avoid division by 0/1 -> Divide/2
  "Flux_ref "/1 -> Divide/1
  Flux_ref/1 -> Switch/3
  wr/1 -> avoid division by 0/1, Switch/2
  Flux/1 -> Sum4/2  "Flux"
  Discrete PI Controller/1(Out) -> Vf/1  "Vf"
  Sum4/1 -> Discrete PI Controller/1(Error)

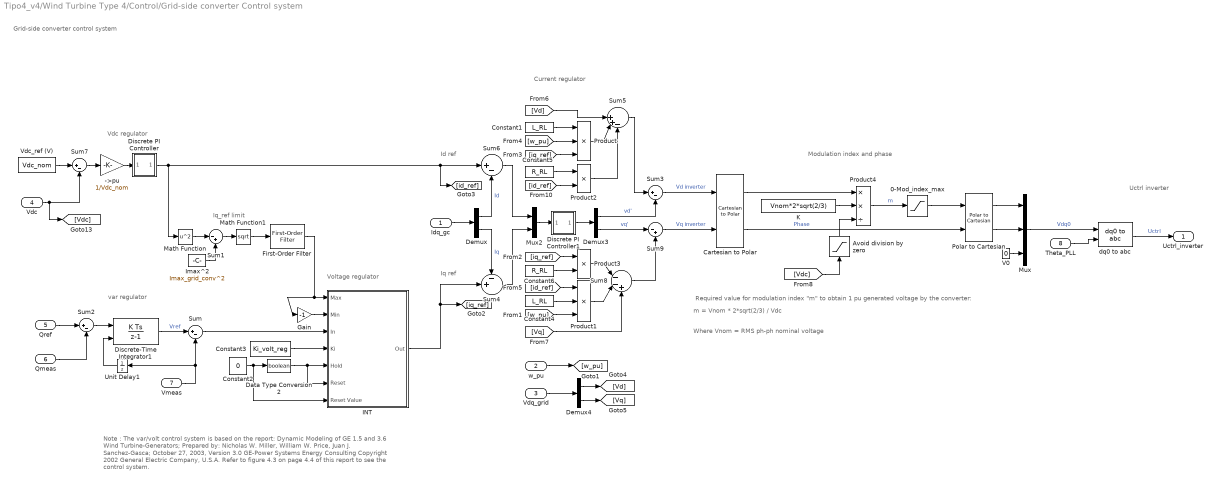
== system Tipo4_v4/Wind Turbine Type 4/Control/Grid-side converter Control system ==
  note: Note :
      | The var/volt control system is based on the report:
      | Dynamic Modeling of GE 1.5 and 3.6 Wind Turbine-Generators;
      | Prepared by: Nicholas W. Miller, William W. Price, Juan J. Sanchez-Gasca;
      | October 27, 2003, Version 3.0
      | GE-Power Systems Energy Consulting
      | Copyright 2002 General Electric Company, U.S.A.
      |
      | Refer to figure 4.3 on page 4.4 of this report to see the control system.
  note: Uctrl inverter
  note: Modulation index and phase
  note: Where Vnom = RMS ph-ph nominal voltage
  note: m = Vnom * 2*sqrt(2/3) / Vdc
  note: Required value for modulation index "m" to obtain 1 pu generated voltage by the converter:
  note: Iq ref
  note: Id ref
  note: Current regulator
  note: Iq_ref limit
  note: Vdc regulator
  note: Voltage regulator
  note: var regulator
  note: Grid-side converter control system
  Idq_gc : Inport
  w_pu : Inport  Port=2
  Vdq_grid : Inport  Port=3
  Vdc : Inport  Port=4
  Qref : Inport  Port=5
  Qmeas : Inport  Port=6
  Vmeas : Inport  Port=7
  Theta_PLL : Inport  Port=8
  ->pu : Gain  Gain=1/Vdc_nom
  0-Mod_index_max : Saturate  UpperLimit=Mod_index_max  LowerLimit=0
  Avoid division by zero : Saturate  UpperLimit=1e6  LowerLimit=1e-6
  Cartesian to Polar : simulink_extras/Transformations/Cartesian to Polar
      settings: SourceProductName=Simulink
  Constant1 : Constant  Value=L_RL
  Constant2 : Constant  Value=0
  Constant3 : Constant  Value=Ki_volt_reg
  Constant4 : Constant  Value=L_RL
  Constant5 : Constant  Value=R_RL
  Constant6 : Constant  Value=R_RL
  Data Type Conversion2 : DataTypeConversion  OutDataTypeStr=boolean
  Demux : Demux  Outputs=2
  Demux3 : Demux  Outputs=2
  Demux4 : Demux  Outputs=2
  Discrete PI Controller : Subsystem  DialogController=POWERSYS.PowerSysDialog  mask(Discrete PI Controller){Kp=Kp_dc, Ki=Ki_dc, Par_Limits=[1 -1]*Imax_grid_conv, Init=0, Ts=Ts}
      mask prompts: Kp "Proportional gain (Kp):"; Ki "Integral gain (Ki):"; Par_Limits "Output limits: [ Upper   Lower ]"; Init "Output initial value:"; Ts "Sample time:"
      mask help: This block implements a discrete PI controller.
      mask init:
      | UpperLimit=Par_Limits(1);
      | LowerLimit=Par_Limits(2);
      | power_initmask();
      mask Help: This block is part of a subset of blocks in the Extras library that does not have documentation associated with it, other than the block mask description.
      mask Display: disp('PI');
  Discrete PI Controller1 : Subsystem  DialogController=POWERSYS.PowerSysDialog  mask(Discrete PI Controller){Kp=Kp_grid_side_cur_reg, Ki=Ki_grid_side_cur_reg, Par_Limits=[1 -1]*Current_reg_output_limit, Init=0, Ts=Ts}
      mask prompts: Kp "Proportional gain (Kp):"; Ki "Integral gain (Ki):"; Par_Limits "Output limits: [ Upper   Lower ]"; Init "Output initial value:"; Ts "Sample time:"
      mask help: This block implements a discrete PI controller.
      mask init:
      | UpperLimit=Par_Limits(1);
      | LowerLimit=Par_Limits(2);
      | power_initmask();
      mask Help: This block is part of a subset of blocks in the Extras library that does not have documentation associated with it, other than the block mask description.
      mask Display: disp('PI');
  Discrete-Time Integrator1 : DiscreteIntegrator  gainval=Ki_var_reg  InitialConditionSource=external  InitialCondition=1  SampleTime=Ts  LimitOutput=on  UpperSaturationLimit=Var_reg_output_hi_limit  LowerSaturationLimit=Var_reg_output_low_limit  ICPrevOutput=DiscIntNeverNeededParam  ICPrevScaledInput=DiscIntNeverNeededParam
  First-Order Filter : powerlib_meascontrol/Filters/First-Order Filter  FilterType=Lowpass  Tc=Iq_ref_limit_time_constant  Ts=Ts  Initialize=on  Vac_Init=[0, 0, 0]  Vdc_Init=Imax_grid_conv  PlotResponse=off  FreqRange="[0,  200,  1]"
      settings: SourceProductName=Simscape Electrical
  Gain : Gain  Gain=-1  SaturateOnIntegerOverflow=on  OutDataTypeStr=Inherit: Same as input  ParamDataTypeStr=Inherit: Same as input
  INT : Subsystem  mask(Integrator  With  External  Dynamic  Limits (Discrete)){}
      mask Display: disp('Discrete-Time\n(Trapezoidal)\nIntegrator\n ')
  Imax^2 : Constant  Value=Imax_grid_conv^2
  K : Constant  Value=Vnom*2*sqrt(2/3)
  Math Function : Math  Operator=square  SaturateOnIntegerOverflow=on
  Math Function1 : Math  Operator=sqrt  SaturateOnIntegerOverflow=on
  Mux : Mux  Inputs=3
  Mux2 : Mux  Inputs=2
  Polar to Cartesian : simulink_extras/Transformations/Polar to Cartesian
      settings: SourceProductName=Simulink  SourceProductBaseCode=SL
  Product : Product  Inputs=3  SaturateOnIntegerOverflow=on  InputSameDT=on  OutDataTypeStr=Inherit: Same as first input
  Product1 : Product  Inputs=3  SaturateOnIntegerOverflow=on  InputSameDT=on  OutDataTypeStr=Inherit: Same as first input
  Product2 : Product  SaturateOnIntegerOverflow=on  InputSameDT=on  OutDataTypeStr=Inherit: Same as first input
  Product3 : Product  SaturateOnIntegerOverflow=on  InputSameDT=on  OutDataTypeStr=Inherit: Same as first input
  Product4 : Product  Inputs=**/  SaturateOnIntegerOverflow=on  InputSameDT=on  OutDataTypeStr=Inherit: Same as first input
  Sum{,2..3,6..7} (5 alike) : Sum  Inputs=|+-  SaturateOnIntegerOverflow=on  InputSameDT=on  OutDataTypeStr=Inherit: Same as first input
  Sum1 : Sum  Inputs=|-+  SaturateOnIntegerOverflow=on  InputSameDT=on  OutDataTypeStr=Inherit: Same as first input
  Sum4 : Sum  Inputs=-+|  SaturateOnIntegerOverflow=on  InputSameDT=on  OutDataTypeStr=Inherit: Same as first input
  Sum5 : Sum  Inputs=||++-  SaturateOnIntegerOverflow=on  InputSameDT=on  OutDataTypeStr=Inherit: Same as first input
  Sum8 : Sum  Inputs=|--+  SaturateOnIntegerOverflow=on  InputSameDT=on  OutDataTypeStr=Inherit: Same as first input
  Sum9 : Sum  Inputs=|-+  SaturateOnIntegerOverflow=on  InputSameDT=on  OutDataTypeStr=Inherit: Same as first input
  Unit Delay1 : UnitDelay  InitialCondition=1  SampleTime=Ts
  V0 : Constant  Value=0
  Vdc_ref (V) : Constant  Value=Vdc_nom
  dq0 to abc : powerlib_meascontrol/Transformations/dq0 to abc  Alignment=90 degrees behind phase A axis
      settings: SourceProductName=Simscape Electrical
  Uctrl_inverter : Outport
  wires:
  Theta_PLL/1 -> dq0 to abc/2
  INT/1(Out) -> [iq_ref], Sum4/2
  Qref/1 -> Sum2/1
  Vdc_ref (V)/1 -> Sum7/1
  Sum8/1 -> Sum9/2
  Sum5/1 -> Sum3/1
  0-Mod_index_max/1 -> Polar to Cartesian/1
  Idq_gc/1 -> Demux/1
  dq0 to abc/1 -> Uctrl_inverter/1  "Uctrl"
  Mux/1 -> dq0 to abc/1  "Vdq0"
  Cartesian to Polar/2 -> Polar to Cartesian/2  "Phase"
  V0/1 -> Mux/3
  Polar to Cartesian/1 -> Mux/1
  Polar to Cartesian/2 -> Mux/2
  Sum9/1 -> Cartesian to Polar/2  "Vq inverter"
  Sum3/1 -> Cartesian to Polar/1  "Vd inverter"
  [Vdc] -> Avoid division by zero/1
  Cartesian to Polar/1 -> Product4/1
  Avoid division by zero/1 -> Product4/3
  K/1 -> Product4/2
  Product4/1 -> 0-Mod_index_max/1  "m"
  [Vd] -> Sum5/1
  [Vq] -> Sum8/3
  Demux4/2 -> [Vq]
  Demux4/1 -> [Vd]
  w_pu/1 -> [w_pu]
  Demux3/2 -> Sum9/1  "vq'"
  Demux3/1 -> Sum3/2  "vd'"
  [id_ref] -> Product1/1
  [iq_ref] -> Product3/1
  [id_ref] -> Product2/2
  [iq_ref] -> Product/3
  [w_pu] -> Product/2
  [w_pu] -> Product1/3
  Sum4/1 -> Mux2/2
  Sum6/1 -> Mux2/1
  Product3/1 -> Sum8/1
  Product2/1 -> Sum5/3
  Product1/1 -> Sum8/2
  Constant6/1 -> Product3/2
  Constant5/1 -> Product2/1
  Product/1 -> Sum5/2
  Demux/1 -> Sum6/2  "Id"
  Demux/2 -> Sum4/1  "Iq"
  Constant1/1 -> Product/1
  Mux2/1 -> Discrete PI Controller1/1(Error)
  Discrete PI Controller1/1(Out) -> Demux3/1
  Constant4/1 -> Product1/2
  First-Order Filter/1 -> INT/1(Max), Gain/1
  Math Function/1 -> Sum1/1
  Imax^2/1 -> Sum1/2
  Sum1/1 -> Math Function1/1
  Math Function1/1 -> First-Order Filter/1
  Unit Delay1/1 -> Discrete-Time Integrator1/2
  Sum2/1 -> Discrete-Time Integrator1/1
  Qmeas/1 -> Sum2/2
  Vmeas/1 -> Sum/2, Unit Delay1/1
  Discrete-Time Integrator1/1 -> Sum/1  "Vref"
  Constant3/1 -> INT/4(Ki)
  Gain/1 -> INT/2(Min)
  Data Type Conversion2/1 -> INT/6(Reset), INT/5(Hold)
  Constant2/1 -> INT/7(Reset Value), Data Type Conversion2/1
  Sum/1 -> INT/3(In)
  Discrete PI Controller/1(Out) -> Sum6/1, [id_ref], Math Function/1
  ->pu/1 -> Discrete PI Controller/1(Error)
  Sum7/1 -> ->pu/1
  Vdq_grid/1 -> Demux4/1
  Vdc/1 -> Sum7/2, [Vdc]
